simulink model "RCseriescircuit"  (R2015a)
settings: Solver=ode3  StartTime=0.0  StopTime=10  RelTol=1e-3
libraries: fl_lib x6, nesl_utility x6
settings Model: Creator=nikos  LastModifiedBy=nikos

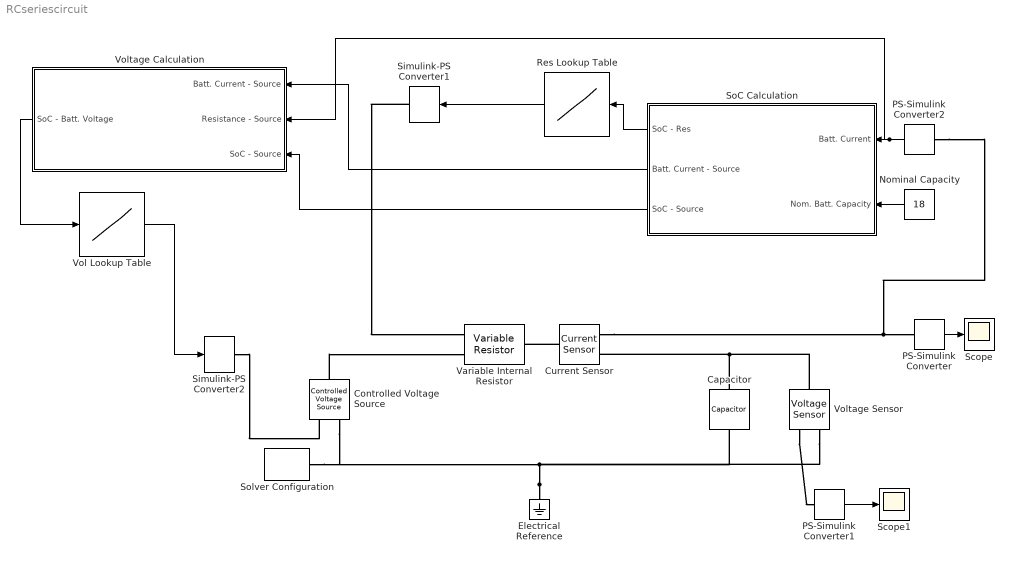
== system RCseriescircuit ==
  Capacitor : fl_lib/Electrical/Electrical Elements/Capacitor  c=10 F  r=1 Ohm  g=0 1/Ohm  i_specify=off  i_priority=High  i=0 A  v_specify=off  v_priority=High  v=0 V  vc_specify=off  vc_priority=High  vc=0 V
  Controlled Voltage Source : fl_lib/Electrical/Electrical Sources/Controlled Voltage Source
  Current Sensor : fl_lib/Electrical/Electrical Sensors/Current Sensor
  Electrical Reference : fl_lib/Electrical/Electrical Elements/Electrical Reference
  Nominal Capacity : Constant  Value=18
  PS-Simulink Converter : nesl_utility/PS-Simulink Converter  PhysicalDomain=network_engine_domain  SubClassName=ps_output  LeftPortType=input  RightPortType=output  PseudoPeriodic=off  Frequencies=[]  Unit=1  AffineConversion=off
  PS-Simulink Converter1 : nesl_utility/PS-Simulink Converter  PhysicalDomain=network_engine_domain  SubClassName=ps_output  LeftPortType=input  RightPortType=output  PseudoPeriodic=off  Frequencies=[]  Unit=1  AffineConversion=off
  PS-Simulink Converter2 : nesl_utility/PS-Simulink Converter  PhysicalDomain=network_engine_domain  SubClassName=ps_output  LeftPortType=input  RightPortType=output  PseudoPeriodic=off  Frequencies=[]  Unit=1  AffineConversion=off
  Res Lookup Table : Lookup_n-D  NumberOfTableDimensions=1  BreakpointsForDimension1=[0, 10, 20, 30, 40, 50, 60, 70, 80, 90, 100]  Table=[0.011448, 0.011038, 0.011281, 0.011236, 0.010959, 0.010714, 0.010698, 0.010712, 0.010917, 0.011304, 0.011603]  InternalRulePriority=Speed  RndMeth=Simplest  InputSameDT=on
  Scope : Scope
      settings: YMin=-0.01  YMax=0.1
  Scope1 : Scope
      settings: YMin=0.55  YMax=0.85
  Simulink-PS Converter1 : nesl_utility/Simulink-PS Converter  PhysicalDomain=network_engine_domain  SubClassName=ps_input  LeftPortType=input  RightPortType=output  PseudoPeriodic=off  Frequencies=[]  NoiseDistribution=none  NoiseParameters=[]  Unit=1  AffineConversion=off  InputFiltering=on  SimscapeFilterOrder=1  InputFilterTimeConstant=0.001  UdotUserProvided=1
  Simulink-PS Converter2 : nesl_utility/Simulink-PS Converter  PhysicalDomain=network_engine_domain  SubClassName=ps_input  LeftPortType=input  RightPortType=output  PseudoPeriodic=off  Frequencies=[]  NoiseDistribution=none  NoiseParameters=[]  Unit=1  AffineConversion=off  InputFiltering=on  SimscapeFilterOrder=1  InputFilterTimeConstant=0.001  UdotUserProvided=1
  SoC Calculation : Subsystem
  Solver Configuration : nesl_utility/Solver Configuration  PhysicalDomain=network_engine_domain  SubClassName=solver  LeftPortType=input  RightPortType=generic  Accelerate=off  Tones=[]  Harmonics=[]  SimulateNoise=off  Profile=off  UseLocalSampling=off  EnableSwitchedLinearOptims=on  FrequencyDomain=off  UseCCode=off  RelTol=0.001  AbsTol=1e-06  MinStep=1e-09  ToWorkspace=off  RevertToSquareIcSolve=off  NumHomotopyIterations=100  DoDC=off  ResidualTolerance=1e-09  UseLocalSolver=off  LocalSolverChoice=NE_BACKWARD_EULER_ADVANCER  LocalSolverSampleTime=0.001  DoFixedCost=off  MaxNonlinIter=3  MaxModeIter=2  LinearAlgebra=Sparse  DelaysMemoryBudget=1024  AutomaticFiltering=on  FilteringTimeConstant=0.001
  Variable Internal Resistor : fl_lib/Electrical/Electrical Elements/Variable Resistor  Rmin=1 Ohm  i_specify=off  i_priority=High  i=0 A  v_specify=off  v_priority=High  v=0 V
  Vol Lookup Table : Lookup_n-D  NumberOfTableDimensions=1  BreakpointsForDimension1=[0,10,20,30,40,50,60,70,80,90,100]  Table=[35.042,35.573,36.009,36.393,36.742,37.121,37.937,38.753,39.7,40.821,41.9299999]  InternalRulePriority=Speed  RndMeth=Simplest  InputSameDT=on
  Voltage Calculation : Subsystem
  Voltage Sensor : fl_lib/Electrical/Electrical Sensors/Voltage Sensor
  wires:
  PS-Simulink Converter/1 -> Scope/1
  PS-Simulink Converter1/1 -> Scope1/1
  PS-Simulink Converter2/1 -> Voltage Calculation/2("Resistance - Source "), SoC Calculation/1("Batt. Current ")
  Nominal Capacity/1 -> SoC Calculation/2("Nom. Batt. Capacity ")
  SoC Calculation/1(SoC - Res) -> Res Lookup Table/1
  Res Lookup Table/1 -> Simulink-PS Converter1/1
  SoC Calculation/2("Batt. Current - Source ") -> Voltage Calculation/1(Batt. Current - Source)
  SoC Calculation/3("SoC - Source ") -> Voltage Calculation/3(SoC - Source)
  Voltage Calculation/1("SoC - Batt. Voltage ") -> Vol Lookup Table/1
  Vol Lookup Table/1 -> Simulink-PS Converter2/1
  connections:
  Electrical Reference/LConn1 -- Controlled Voltage Source/RConn2 -- Solver Configuration/RConn1 -- Voltage Sensor/RConn2 -- Capacitor/RConn1
  Current Sensor/LConn1 -- Variable Internal Resistor/RConn1
  Current Sensor/RConn1 -- PS-Simulink Converter2/LConn1 -- PS-Simulink Converter/LConn1
  Voltage Sensor/LConn1 -- Capacitor/LConn1 -- Current Sensor/RConn2
  Voltage Sensor/RConn1 -- PS-Simulink Converter1/LConn1
  Controlled Voltage Source/LConn1 -- Variable Internal Resistor/LConn2
  Simulink-PS Converter1/RConn1 -- Variable Internal Resistor/LConn1
  Simulink-PS Converter2/RConn1 -- Controlled Voltage Source/RConn1

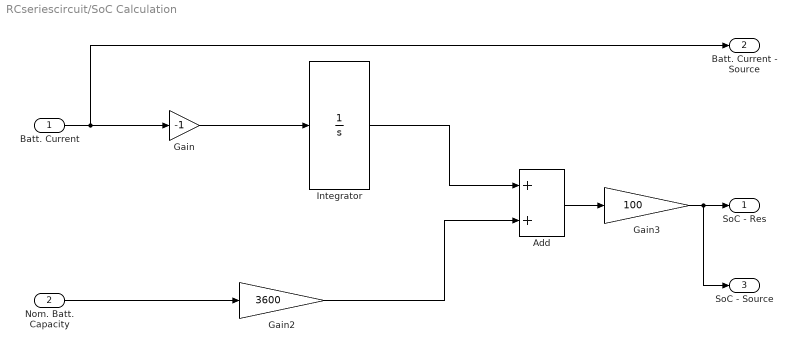
== system RCseriescircuit/SoC Calculation ==
  "Batt. Current " : Inport
  "Nom. Batt. Capacity " : Inport  Port=2  OutMin=0  OutMax=100
  Add : Sum
  Gain : Gain  Gain=-1
  Gain2 : Gain  Gain=3600
  Gain3 : Gain  Gain=100
  Integrator : Integrator
  SoC - Res : Outport
  "Batt. Current - Source " : Outport  Port=2
  "SoC - Source " : Outport  Port=3
  wires:
  "Batt. Current "/1 -> "Batt. Current - Source "/1, Gain/1
  Gain/1 -> Integrator/1
  "Nom. Batt. Capacity "/1 -> Gain2/1
  Gain2/1 -> Add/2
  Add/1 -> Gain3/1
  Integrator/1 -> Add/1
  Gain3/1 -> "SoC - Source "/1, SoC - Res/1

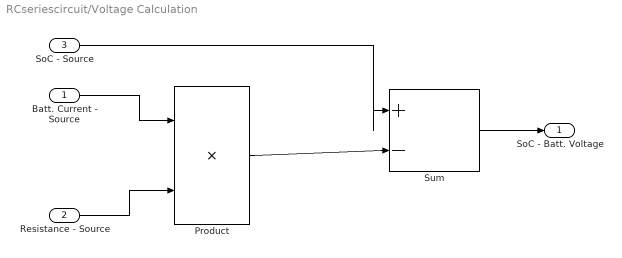
== system RCseriescircuit/Voltage Calculation ==
  Batt. Current - Source : Inport
  "Resistance - Source " : Inport  Port=2
  SoC - Source : Inport  Port=3
  Product : Product
  Sum : Sum  Inputs=|+-
  "SoC - Batt. Voltage " : Outport
  wires:
  Product/1 -> Sum/2
  Batt. Current - Source/1 -> Product/1
  "Resistance - Source "/1 -> Product/2
  SoC - Source/1 -> Sum/1
  Sum/1 -> "SoC - Batt. Voltage "/1
